simulink model "experimental_results"  (Simulink 10.2)
settings: Solver=ode1  StartTime=0.0  StopTime=60  FixedStep=0.002  RelTol=1e-3  EnableMultiTasking=on
PreLoadFcn:
  | quanser_aero_lqr
undefined symbols (not defined in the file or in its folder): HIL, qc_get_step_size
libraries: quarc_library x7
(part 2 of 2)

== matlab function DTEKF ==
  data: xbark input double; measurements input double; xbark1 output double; u input double; Pbark input double; Pbark1 output double
function [xbark1, Pbark1] = DTExtendedKalmanFilter(xbark, measurements, u, Pbark)
    h = 0.002; % time step
 
    R = diag([2.36e-6; 5.8974e-07]);
    Q = diag([0; 0; 1; 1]);
    H = [eye(2), zeros(2)];
    
    K = Pbark * H' / (H * Pbark * H' + R);
    xhat = xbark + K * (measurements - H * xbark);
    Phat = (eye(4) - K * H) * Pbark * (eye(4) - K * H)' + K * R * K';

    theta = xhat(1);
    psi = xhat(2);
    thetadot = xhat(3);
    psidot = xhat(4);

    utilde = u.^2;
    utilde1 = utilde(1);
    utilde2 = utilde(2);
    
    % parameters
    g = 9.81;
    dt = 0.158;
    me = 0.2;
    dx = 0.02;
    
    ry = 0.02;
    my = 0.526;
    
    mpa = 0.146;
    lt = 0.165;
    mmt = 0.089;
    mtt = 0.089;
    mtc = 0.280;
    mrod = mmt + mtt + mtc;
    
    Ibyy = 2*mpa*dt^2 + 2*me*dt^2 + me*dx^2 + 1/12*mrod*lt^2;
    Ifyzz = 1/2*my*ry^2;

    kt = 0.042;
    km = 0.042;
    kd = 1e-5;
    Rm = 8.4;
    
    Komega = kt / (kt * km + kd * Rm);
    
    Kmtheta = 1.58e-6;
    Kttheta = 1.35e-6;
    Kmpsi = Kttheta;
    Ktpsi = Kmtheta; 
    
    d1 = 0.00711;
    d2 = 0.0220;
    
    F = [
                                                                                                                                                                                                                                                                                                                                                                                           0, 0,                                                                 1,                                                              0;
                                                                                                                                                                                                                                                                                                                                                                                           0, 0,                                                                 0,                                                              1;
                                                                                                                                                                                                                                                                                                                             -(Ibyy*(2*cos(theta)^2 - 1)*psidot^2 + dx*g*me*cos(theta))/Ibyy, 0,                                                          -d1/Ibyy,                                           -psidot*sin(2*theta);
        (4*Ibyy*psidot*thetadot*(2*cos(theta)^2 - 1) + 2*Kmpsi*Komega^2*dt*utilde1*sin(theta) - 2*Komega^2*Ktpsi*dt*utilde2*sin(theta))/(Ibyy + 2*Ifyzz + Ibyy*(2*cos(theta)^2 - 1)) - (2*Ibyy*cos(theta)*sin(theta)*(d2*psidot + Kmpsi*Komega^2*dt*utilde1*cos(theta) - Komega^2*Ktpsi*dt*utilde2*cos(theta) - 2*Ibyy*psidot*thetadot*cos(theta)*sin(theta)))/(Ibyy*cos(theta)^2 + Ifyzz)^2, 0, (2*Ibyy*psidot*cos(theta)*sin(theta))/(Ibyy*cos(theta)^2 + Ifyzz), -(d2 - Ibyy*thetadot*sin(2*theta))/(Ibyy*cos(theta)^2 + Ifyzz);
    ];

%     h = H * xhat;

    M = [
        Ibyy, 0;
        0, Ifyzz + Ibyy * cos(theta)^2;
    ];
    C = [
        0, Ibyy * psidot * cos(theta)*sin(theta);
        0, -2*Ibyy * thetadot * cos(theta)*sin(theta);
    ];
    gvec = [
        dx * g * me * sin(theta);
        0;
    ];
    B = Komega^2 * dt * [
        Kmtheta, Kttheta;
        -Kmpsi * cos(theta), Ktpsi * cos(theta);
    ];
    D = [
        d1, 0;
        0, d2;
    ];
    qdot = [
        thetadot;
        psidot;
    ];
    
    f = [
        qdot;
        M \ (B*utilde - C*qdot - gvec - D*qdot);
    ];
    
    xbark1 = xhat + h * f;
    Pbark1 = (eye(4) + h * F) * Phat * (eye(4) + h * F)' + h^2 * Q;
end

== matlab function OLD CANCELLATION ==
  data: v input double; states input double; u output double
function u = NonlinearityCancellation(v, states)
    theta = states(1);
    psi = states(2);
    thetadot = states(3);
    psidot = states(4);
    
    % parameters
    g = 9.81;
    dt = 0.158;
    me = 0.2;
    dx = 0.02;
    
    ry = 0.02;
    my = 0.526;
    
    mpa = 0.146;
    lt = 0.165;
    mmt = 0.089;
    mtt = 0.089;
    mtc = 0.280;
    mrod = mmt + mtt + mtc;
    
    kt = 0.042;
    km = 0.042;
    kd = 1e-5;
    Rm = 8.4;
    
    Ibyy = 2*mpa*dt^2 + 2*me*dt^2 + me*dx^2 + 1/12*mrod*lt^2;
    Ifyzz = 1/2*my*ry^2;
    
    M = [
        Ibyy, 0;
        0, Ifyzz + Ibyy * cos(theta)^2;
    ];
    C = [
        0, Ibyy * psidot * cos(theta)*sin(theta);
        0, -2*Ibyy * thetadot * cos(theta)*sin(theta);
    ];
    gvec = [
        dx * g * me * sin(theta);
        0;
    ];
    
    Kmtheta = 1.58e-6;
    Kttheta = 1.35e-6;
    Kmpsi = Kttheta;
    Ktpsi = Kmtheta; 
%     Kmpsi = 2.33e-7;
%     Ktpsi = 3.42e-7;
    
    K_omega = kt / (kt * km + kd * Rm);
%     K_omega = 17.38;
    
    B = K_omega^2 * dt * [
        Kmtheta, Kttheta;
        -Kmpsi * cos(theta), Ktpsi * cos(theta);
    ];

    D = [
        0.00711, 0;
        0, 0.0220;
    ];

    q = [
        theta;
        psi;
    ];
    qdot = [
        thetadot;
        psidot;
    ];

    utilde = B \ (M*v + C * qdot + D * qdot + gvec);
    u = sign(utilde) .* sqrt(abs(utilde));
end

== matlab function Double Integrator Controller/Terminal Sliding Mode Controller (yaw) ==
  data: e input double; u output double; edot input double; kappa input double; rho input double; epsilon input double
function u = TerminalSlidingModeController(e, edot, kappa, rho, epsilon)
    % u = TerminalSlidingModeController(e, edot, kappa, rho, epsilon) 
    % computes the feedback control for a terminal sliding mode controller 
    % given the positive parameters kappa, rho and epsilon.
    %
    % Author:   Finn F. Sandvand
    % Date:     15th Jun 2025
    % Revisions: 

    sign_e = e / (abs(e) + epsilon);
    sigma = edot + kappa * sign(e) * sqrt(abs(e));
    sign_sigma = sigma / (abs(sigma) + epsilon);
    
    mu = 0.5 * kappa^2 + rho;
    u = 0.5 * kappa^2 * sign_e - mu * sign_sigma;
end

== matlab function Double Integrator Controller/Terminal Sliding Mode Controller (pitch) ==
  data: e input double; u output double; edot input double; kappa input double; rho input double; epsilon input double
function u = TerminalSlidingModeController(e, edot, kappa, rho, epsilon)
    % u = TerminalSlidingModeController(e, edot, kappa, rho, epsilon) 
    % computes the feedback control for a terminal sliding mode controller 
    % given the positive parameters kappa, rho and epsilon.
    %
    % Author:   Finn F. Sandvand
    % Date:     15th Jun 2025
    % Revisions: 

    sign_e = e / (abs(e) + epsilon);
    sigma = edot + kappa * sign_e * sqrt(abs(e));
    sign_sigma = sigma / (abs(sigma) + epsilon);
    
    mu = 0.5 * kappa^2 + rho;
    u = 0.5 * kappa^2 * sign_e - mu * sign_sigma;
end
